simulink library "CMGlibrary"  (R2019b)
settings: Solver=VariableStepAuto  StartTime=0.0  StopTime=10.0  RelTol=1e-3
values from neighbouring files (symbols this model uses):
  angleOffset = 0 *pi/180    (= 0)    [CMGParams.m]
  CMGInertia_z = 3/4*CMGmass*(CMGr)^2    (= 0.0012)    [CMGParams.m]
  CMGmass = 1    [CMGParams.m]
  deltaLegAngleThr = 8*pi/180    (= 0.13962634016)    [CMGParams.m]
  highpassbandFreq = 10    [CMGParams.m]
  KdGammaReset = 6000    [CMGParams.m]
  KiGamma = 1    [CMGParams.m]
  KpGamma = 10    [CMGParams.m]
  KpGammaReset = 30000    [CMGParams.m]
  legAngleSpeedMax = 10    [CMGParams.m]
  lowpassbandFreq = 80    [CMGParams.m]
  maxGMangle = 60 *pi/180    (= 1.0471975512)    [CMGParams.m]
  maxGMTorque = 15    [CMGParams.m]
  maxTflywheelmotor = 1.83E-3    (= 0.00183)    [CMGParams.m]
  N = 1.5    [BodyMechParams.m]    (also in cmaes.m = size(x,1); mergeCompareEnergyCosts.m = {S.name})
  omegaRef = 2100    [CMGParams.m]
  RkneeExtendGain = 25000    [CMGParams.m]
  RkneeFlexPosGain = 6    [CMGParams.m]
  RkneeFlexSpeedGain = 6    [CMGParams.m]
  RkneeStopGain = 12000    [CMGParams.m]
  RlegAngleFilter = 100    [CMGParams.m]
  s = x(1:N-1,:).^2 + x(2:N,:).^2    [cmaes.m]
  shankLength = shankLength - ankle_height/2    (= 0.46)    [BodyMechParams.m]
  TargetLegAngleTripFlex = 2/3*pi    (= 2.09439510239)    [CMGParams.m]
  thighLength = thighLength - ankle_height/2    (= 0.46)    [BodyMechParams.m]
  tripDetectThreshold = -600    [CMGParams.m]
  X = contains(N,'compareEnergyCost') .* ~contains(N,'total') .* ~contains(N,'Total')    [mergeCompareEnergyCosts.m]
  zeroOrderHoldTs = 1/1000    (= 0.001)    [CMGParams.m]
undefined symbols (not defined in the file or in its folder): kneeExtendGain, kneeFlexPosGain, kneeFlexSpeedGain, kneeStopGain, legAngleFilter, legLengthClr, RdeltaLegAngleThr, RlegLengthClr, Y, Z
libraries: sm_lib x11, nesl_utility x11, dspfdesign x6, simulink x5, $bdroot x1, dspsigops x1
settings Model: Creator=sup-gjtimmers  LastModifiedBy=Nathan

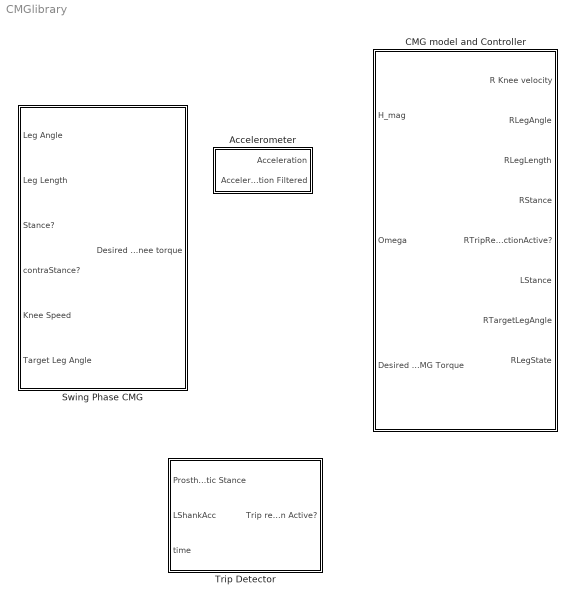
== system CMGlibrary ==
  Accelerometer : Subsystem  mask{zoh_sampletime=zeroOrderHoldTs, lowpasswp=lowpassbandFreq, highpasswp=highpassbandFreq}
      mask prompts: zoh_sampletime "Zero-order hold sample time (s)"; lowpasswp "Lowpass passband frequency (Hz)"; highpasswp "Highpass passband frequency (Hz)"
  CMG model and Controller : Subsystem  mask{KpGamma=KpGamma, KiGamma=KiGamma, legAngleFilter=RlegAngleFilter, kneeFlexSpeedGain=RkneeFlexSpeedGain, kneeFlexPosGain=RkneeFlexPosGain, kneeStopGain=RkneeStopGain, kneeExtendGain=RkneeExtendGain, legLengthClr=RlegLengthClr, TargetLegAngleTripFlex=TargetLegAngleTripFlex, deltaLegAngleThr=RdeltaLegAngleThr, legAngleSpeedMax=legAngleSpeedMax}
      mask prompts: KpGamma "Proportional Gain Gamma ( Nm/(rad/s) )"; KiGamma "Integral Gain Gamma (Nm/rad)"
  Swing Phase CMG : Subsystem  mask{legAngleFilter=legAngleFilter, kneeFlexSpeedGain=kneeFlexSpeedGain, kneeFlexPosGain=kneeFlexPosGain, kneeStopGain=kneeStopGain, kneeExtendGain=kneeExtendGain, legLengthClr=legLengthClr, TargetLegAngleTripFlex=TargetLegAngleTripFlex, deltaLegAngleThr=deltaLegAngleThr, legAngleSpeedMax=legAngleSpeedMax}
  Trip Detector : Subsystem  mask{tripThreshold=tripDetectThreshold}
      mask prompts: tripThreshold "Trip threshold (m/s^2)"

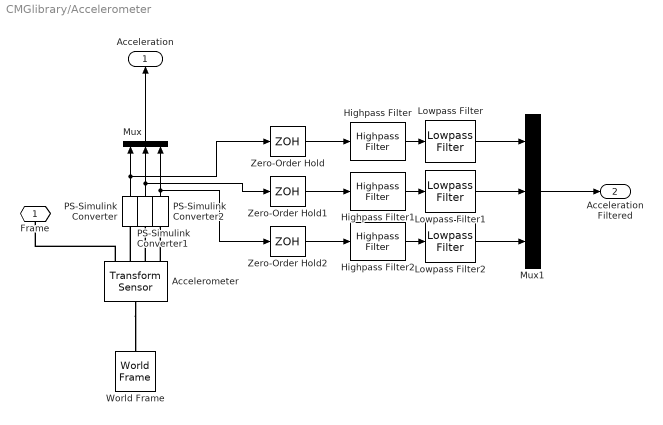
== system CMGlibrary/Accelerometer ==
  Accelerometer : sm_lib/Frames and Transforms/Transform Sensor  MeasurementFrame=World  SenseAngle=off  SenseAxis=off  SenseAngle1=off  SenseAngle2=off  SenseAngle3=off  SenseQ=off  SenseR=off  SenseOmegaX=off  SenseOmegaY=off  SenseOmegaZ=off  SenseOmega1=off  SenseOmega2=off  SenseOmega3=off  SenseQDot=off  SenseRDot=off  SenseAlphaX=off  SenseAlphaY=off  SenseAlphaZ=off  SenseAlpha1=off  SenseAlpha2=off  SenseAlpha3=off  SenseQDDot=off  SenseRDDot=off  SenseX=off  SenseY=off  SenseZ=off  SenseRad=off  SenseAzim=off  SenseDist=off  SenseInc=off  SenseXDot=off  SenseYDot=off  SenseZDot=off  SenseRadDot=off  SenseAzimDot=off  SenseDistDot=off  SenseIncDot=off  SenseXDDot=on  SenseYDDot=on  SenseZDDot=on  SenseRadDDot=off  SenseAzimDDot=off  SenseDistDDot=off  SenseIncDDot=off
  Highpass Filter : dspfdesign/Highpass Filter  FilterType=IIR  DesignForMinimumOrder=off  FilterOrder=2  StopbandFrequency=2.5  PassbandFrequency=highpasswp  StopbandAttenuation=60  PassbandRipple=0.1  InheritSampleRate=on  SampleRate=1000  SimulateUsing=Interpreted execution  roundingMode=Floor  coeffsDataTypeStr=fixdt(1,16)
      settings: SourceProductName=DSP System Toolbox
  Highpass Filter1 : dspfdesign/Highpass Filter  FilterType=IIR  DesignForMinimumOrder=off  FilterOrder=2  StopbandFrequency=2.5  PassbandFrequency=highpasswp  StopbandAttenuation=60  PassbandRipple=0.1  InheritSampleRate=on  SampleRate=1000  SimulateUsing=Interpreted execution  roundingMode=Floor  coeffsDataTypeStr=fixdt(1,16)
      settings: SourceProductName=DSP System Toolbox
  Highpass Filter2 : dspfdesign/Highpass Filter  FilterType=IIR  DesignForMinimumOrder=off  FilterOrder=2  StopbandFrequency=2.5  PassbandFrequency=highpasswp  StopbandAttenuation=60  PassbandRipple=0.1  InheritSampleRate=on  SampleRate=1000  SimulateUsing=Interpreted execution  roundingMode=Floor  coeffsDataTypeStr=fixdt(1,16)
      settings: SourceProductName=DSP System Toolbox
  Lowpass Filter : dspfdesign/Lowpass Filter  FilterType=IIR  DesignForMinimumOrder=off  FilterOrder=2  PassbandFrequency=lowpasswp  StopbandFrequency=41  PassbandRipple=0.2  StopbandAttenuation=80  InheritSampleRate=on  SampleRate=1000  SimulateUsing=Interpreted execution  roundingMode=Floor  coeffsDataTypeStr=fixdt(1,16)
  Lowpass Filter1 : dspfdesign/Lowpass Filter  FilterType=IIR  DesignForMinimumOrder=off  FilterOrder=2  PassbandFrequency=lowpasswp  StopbandFrequency=41  PassbandRipple=0.2  StopbandAttenuation=80  InheritSampleRate=on  SampleRate=1000  SimulateUsing=Interpreted execution  roundingMode=Floor  coeffsDataTypeStr=fixdt(1,16)
  Lowpass Filter2 : dspfdesign/Lowpass Filter  FilterType=IIR  DesignForMinimumOrder=off  FilterOrder=2  PassbandFrequency=lowpasswp  StopbandFrequency=41  PassbandRipple=0.2  StopbandAttenuation=80  InheritSampleRate=on  SampleRate=1000  SimulateUsing=Interpreted execution  roundingMode=Floor  coeffsDataTypeStr=fixdt(1,16)
  Mux : Mux  Inputs=3
  Mux1 : Mux  Inputs=3
  PS-Simulink Converter : nesl_utility/PS-Simulink Converter  PhysicalDomain=network_engine_domain  SubClassName=ps_output  LeftPortType=input  RightPortType=output  PseudoPeriodic=off  Frequencies=[]  Unit=m/s^ 2  AffineConversion=off
  PS-Simulink Converter1 : nesl_utility/PS-Simulink Converter  PhysicalDomain=network_engine_domain  SubClassName=ps_output  LeftPortType=input  RightPortType=output  PseudoPeriodic=off  Frequencies=[]  Unit=m/s^ 2  AffineConversion=off
  PS-Simulink Converter2 : nesl_utility/PS-Simulink Converter  PhysicalDomain=network_engine_domain  SubClassName=ps_output  LeftPortType=input  RightPortType=output  PseudoPeriodic=off  Frequencies=[]  Unit=m/s^ 2  AffineConversion=off
  World Frame : sm_lib/Frames and Transforms/World Frame
  Zero-Order Hold : ZeroOrderHold  SampleTime=zoh_sampletime
  Zero-Order Hold1 : ZeroOrderHold  SampleTime=zoh_sampletime
  Zero-Order Hold2 : ZeroOrderHold  SampleTime=zoh_sampletime
  Frame : PMIOPort  Side=Left
  Acceleration : Outport
  Acceleration Filtered : Outport  Port=2
  wires:
  PS-Simulink Converter1/1 -> Zero-Order Hold1/1, Mux/2
  PS-Simulink Converter/1 -> Mux/1, Zero-Order Hold/1
  Mux/1 -> Acceleration/1
  PS-Simulink Converter2/1 -> Zero-Order Hold2/1, Mux/3
  Zero-Order Hold/1 -> Highpass Filter/1
  Highpass Filter/1 -> Lowpass Filter/1
  Highpass Filter1/1 -> Lowpass Filter1/1
  Zero-Order Hold1/1 -> Highpass Filter1/1
  Zero-Order Hold2/1 -> Highpass Filter2/1
  Highpass Filter2/1 -> Lowpass Filter2/1
  Lowpass Filter2/1 -> Mux1/3
  Lowpass Filter1/1 -> Mux1/2
  Lowpass Filter/1 -> Mux1/1
  Mux1/1 -> Acceleration Filtered/1
  connections:
  Accelerometer/LConn1 -- World Frame/RConn1
  Accelerometer/RConn3 -- PS-Simulink Converter1/LConn1
  Accelerometer/RConn1 -- Frame/RConn1
  Accelerometer/RConn2 -- PS-Simulink Converter/LConn1
  Accelerometer/RConn4 -- PS-Simulink Converter2/LConn1

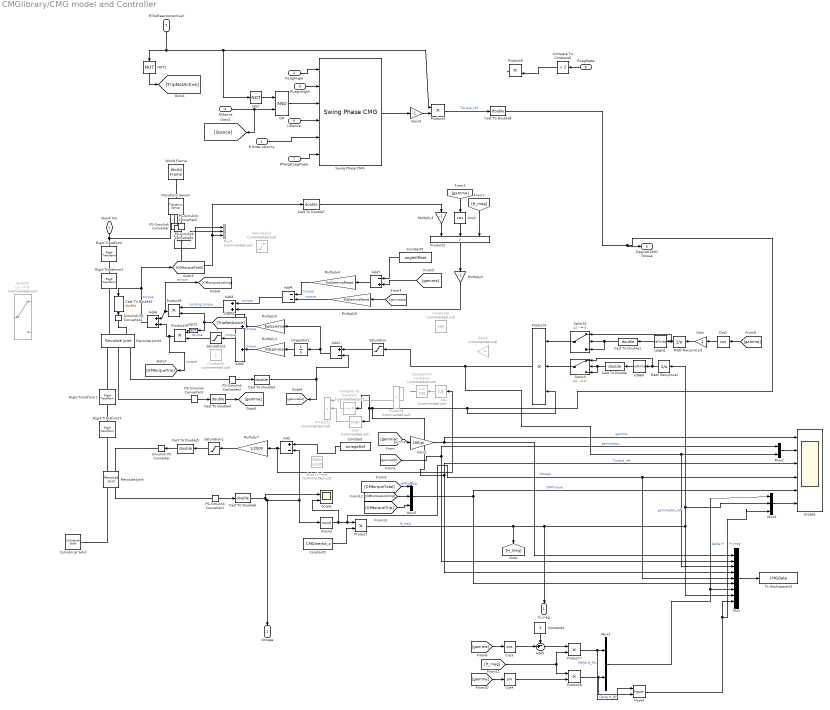
== system CMGlibrary/CMG model and Controller ==
  R Knee velocity : Inport
  RLegAngle : Inport  Port=2
  RLegLength : Inport  Port=3
  RStance : Inport  Port=4
  RTripReactionActive? : Inport  Port=5
  LStance : Inport  Port=6
  RTargetLegAngle : Inport  Port=7
  RLegState : Inport  Port=8
  Abs : Abs  Commented=on  ZeroCross=off
  Add : Sum  Inputs=+-
  Add1 : Sum  Inputs=+-
  Add2 : Sum
  Add3 : Sum
  Add4 : Sum  Inputs=--
  Add5 : Sum  Inputs=-+|
  Add6 : Sum
  Add7 : Sum  Inputs=-+
  Cast To Double{,1..8} (9 alike) : DataTypeConversion  OutDataTypeStr=double  LockScale=on
  Compare To Constant : simulink/Logic and Bit Operations/Compare To Constant  Commented=on  relop=~=  const=0  OutDataTypeStr=boolean  ZeroCross=off
  Compare To Constant1 : simulink/Logic and Bit Operations/Compare To Constant  Commented=on  relop=<=  const=100  OutDataTypeStr=boolean  ZeroCross=off
  Compare To Constant2 : simulink/Logic and Bit Operations/Compare To Constant  relop=<  const=2  OutDataTypeStr=boolean
  Constant : Constant  Value=omegaRef
  Constant1 : Constant  Value=CMGInertia_z
  Constant2 : Constant  Commented=on  Value=150
  Constant3 : Constant  Commented=on
  Constant4 : Constant
  Constant5 : Constant  Value=angleOffset
  Cos1 : Trigonometry  Operator=cos  OutputSignalType=real
  Cos2 : Trigonometry  Operator=cos  OutputSignalType=real
  Cos3 : Trigonometry  Operator=cos  OutputSignalType=real
  Cos4 : Trigonometry  OutputSignalType=real
  Cylindrical Solid : sm_lib/Body Elements/Cylindrical Solid  GraphicAmbientColor=[0.15 0.15 0.15 1.0]  BasedOnType=Mass  CenterOfMass=[0 0 0]  CenterOfMassUnits=m  GraphicDiffuseColor=[0.5 0.5 0.5]  CylinderLength=CMGt  CylinderLengthUnits=m  CylinderRadius=CMGr  CylinderRadiusUnits=m  Density=1000000  DensityUnits=kg/m^3  DoExposeReferenceFrame=on  GraphicEmissiveColor=[0.0 0.0 0.0 1.0]  ExportEntireGeometry=off  SerializedFrames=<Frames/>  MarkerShape=Sphere  MarkerSize=10  GraphicType=FromGeometry  InertiaType=Custom  Mass=CMGmass  MassUnits=kg  MomentsOfInertia=CMGInertia  MomentsOfInertiaUnits=kg*m^2  GraphicOpacity=1.0  ProductsOfInertia=[0 0 0]  ProductsOfInertiaUnits=kg*m^2  GraphicShininess=75  GraphicSpecularColor=[0.5 0.5 0.5 1.0]  GraphicVisPropType=SimpleVisualProperties
  Gain : Gain
  Gain1 : Gain  Commented=on  Gain=4
  Gain2 : Gain  Gain=180/pi
  Gain3 : Gain  Gain=-1
  Hypot : Math  Operator=hypot  SignedPower=off  SaturateOnIntegerOverflow=on
  Integrator1 : Integrator
  IsNaN : RelationalOperator  Operator=isFinite  OutDataTypeStr=boolean  RndMeth=Simplest
  IsNaN1 : RelationalOperator  Operator=isFinite  OutDataTypeStr=boolean  RndMeth=Simplest
  Math Reciprocal : Math  Operator=reciprocal  SaturateOnIntegerOverflow=on
  Math Reciprocal1 : Math  Operator=reciprocal  SaturateOnIntegerOverflow=on
  Multiply1 : Gain  Gain=KiGamma
  Multiply2 : Gain  Gain=-1
  Multiply3 : Gain  Gain=-1
  Multiply4 : Gain  Gain=KpGammaReset
  Multiply5 : Gain  Gain=KpGamma
  Multiply6 : Gain  Gain=KdGammaReset
  Multiply7 : Gain  Gain=1/2000
  Mux : Mux  Inputs=9
  Mux1 : Mux  Commented=on  Inputs=3
  Mux2 : Mux  Inputs=2
  Mux3 : Mux  Inputs=2
  Mux4 : Mux  Inputs=3
  Mux5 : Mux  Inputs=3
  NOT : Logic  Operator=NOT  IconShape=distinctive  AllPortsSameDT=off  OutDataTypeStr=boolean
  NOT1 : Logic  Operator=NOT  IconShape=distinctive  AllPortsSameDT=off  OutDataTypeStr=boolean
  NOT2 : Logic  Operator=NOT  IconShape=distinctive  AllPortsSameDT=off  OutDataTypeStr=boolean
  OR : Logic  AllPortsSameDT=off  OutDataTypeStr=boolean
  PS-Simulink Converter{,1,4..5} (4 alike) : nesl_utility/PS-Simulink Converter  PhysicalDomain=network_engine_domain  SubClassName=ps_output  LeftPortType=input  RightPortType=output  PseudoPeriodic=off  Frequencies=[]  Unit=inherit  AffineConversion=off
  PS-Simulink Converter2 : nesl_utility/PS-Simulink Converter  PhysicalDomain=network_engine_domain  SubClassName=ps_output  LeftPortType=input  RightPortType=output  PseudoPeriodic=off  Frequencies=[]  Unit=rad/s  AffineConversion=off
  PS-Simulink Converter3 : nesl_utility/PS-Simulink Converter  PhysicalDomain=network_engine_domain  SubClassName=ps_output  LeftPortType=input  RightPortType=output  PseudoPeriodic=off  Frequencies=[]  Unit=rad  AffineConversion=off
  Product{,5..10} (7 alike) : Product
  Product1 : Product  Commented=on  Inputs=3
  Product2 : Product  Inputs=3
  Product3 : Product  Commented=on
  Product4 : Product  Inputs=***
  Rate Limiter : RateLimiter  Commented=on  RisingSlewLimit=100000  FallingSlewLimit=-100000  SampleTimeMode=inherited
  Revolute Joint : sm_lib/Joints/Revolute Joint  JointMode=Normal  SenseConstraintForce=off  SenseConstraintForceX=off  SenseConstraintForceY=off  SenseConstraintForceZ=off  SenseConstraintTorque=off  SenseConstraintTorqueX=off  SenseConstraintTorqueY=off  SenseConstraintTorqueZ=off  SenseTotalForce=off  SenseTotalForceX=off  SenseTotalForceY=off  SenseTotalForceZ=off  SenseTotalTorque=off  SenseTotalTorqueX=off  SenseTotalTorqueY=off  SenseTotalTorqueZ=off  CompositeWrenchDir=FollowerOnBase  CompositeWrenchFrame=BaseFrame  EquilibriumPosition=0  EquilibriumPositionUnits=deg  SpringStiffness=0  SpringStiffnessUnits=N*m/deg  DampingCoefficient=0  DampingCoefficientUnits=N*m/(deg/s)  TorqueActuationMode=InputTorque  MotionActuationMode=ComputedMotion  SensePosition=off  SenseVelocity=on  SenseAcceleration=off  SenseTorqueForce=off  SenseLowerLimitTorqueForce=off  SenseUpperLimitTorqueForce=off  LowerLimitSpecify=off  LowerLimitBound=-90  LowerLimitBoundUnits=deg  LowerLimitStiffness=1e4  LowerLimitStiffnessUnits=N*m/deg  LowerLimitDamping=10  LowerLimitDampingUnits=N*m/(deg/s)  LowerLimitTransitionRegionWidth=0.1  LowerLimitTransitionRegionWidthUnits=deg  UpperLimitSpecify=off  UpperLimitBound=90  UpperLimitBoundUnits=deg  UpperLimitStiffness=1e4  UpperLimitStiffnessUnits=N*m/deg  UpperLimitDamping=10  UpperLimitDampingUnits=N*m/(deg/s)  UpperLimitTransitionRegionWidth=0.1  UpperLimitTransitionRegionWidthUnits=deg  PositionTargetSpecify=off  PositionTargetPriority=High  PositionTargetValue=0  PositionTargetValueUnits=deg  VelocityTargetSpecify=on  VelocityTargetPriority=High  VelocityTargetValue=omegaRef  VelocityTargetValueUnits=rad/s
  Revolute Joint2 : sm_lib/Joints/Revolute Joint  JointMode=Normal  SenseConstraintForce=off  SenseConstraintForceX=off  SenseConstraintForceY=off  SenseConstraintForceZ=off  SenseConstraintTorque=off  SenseConstraintTorqueX=off  SenseConstraintTorqueY=off  SenseConstraintTorqueZ=off  SenseTotalForce=off  SenseTotalForceX=off  SenseTotalForceY=off  SenseTotalForceZ=off  SenseTotalTorque=off  SenseTotalTorqueX=off  SenseTotalTorqueY=off  SenseTotalTorqueZ=off  CompositeWrenchDir=FollowerOnBase  CompositeWrenchFrame=BaseFrame  EquilibriumPosition=0  EquilibriumPositionUnits=deg  SpringStiffness=0  SpringStiffnessUnits=N*m/deg  DampingCoefficient=0  DampingCoefficientUnits=N*m/(deg/s)  TorqueActuationMode=InputTorque  MotionActuationMode=ComputedMotion  SensePosition=on  SenseVelocity=on  SenseAcceleration=off  SenseTorqueForce=off  SenseLowerLimitTorqueForce=off  SenseUpperLimitTorqueForce=off  LowerLimitSpecify=on  LowerLimitBound=-maxGMangle  LowerLimitBoundUnits=rad  LowerLimitStiffness=1e4  LowerLimitStiffnessUnits=N*m/deg  LowerLimitDamping=10  LowerLimitDampingUnits=N*m/(deg/s)  LowerLimitTransitionRegionWidth=0.1  LowerLimitTransitionRegionWidthUnits=deg  UpperLimitSpecify=on  UpperLimitBound=maxGMangle  UpperLimitBoundUnits=rad  UpperLimitStiffness=1e4  UpperLimitStiffnessUnits=N*m/deg  UpperLimitDamping=10  UpperLimitDampingUnits=N*m/(deg/s)  UpperLimitTransitionRegionWidth=0.1  UpperLimitTransitionRegionWidthUnits=deg  PositionTargetSpecify=on  PositionTargetPriority=High  PositionTargetValue=angleOffset  PositionTargetValueUnits=rad  VelocityTargetSpecify=on  VelocityTargetPriority=High  VelocityTargetValue=0  VelocityTargetValueUnits=rad/s
  Rigid Transform : sm_lib/Frames and Transforms/Rigid Transform  TranslationMethod=Cartesian  TranslationStandardOffset=0  TranslationLengthUnit=m  TranslationStandardAxis=+Z  TranslationCartesianOffset=[0 -0.015 0]  TranslationROffset=0  TranslationROffsetUnits=m  TranslationZOffset=0  TranslationZOffsetUnits=m  TranslationThetaOffset=0  TranslationThetaOffsetUnits=deg  RotationMethod=None  RotationAngleUnits=deg  RotationStandardAxis=+Z  RotationAngle=0.0  RotationArbitraryAxis=[0 0 1]  FollAlignAxisA=+X  BaseAlignAxisA=+Y  FollAlignAxisB=+Y  BaseAlignAxisB=+Z  RotationSequenceAxes=FollowerAxes  RotationSequence=XYX  RotationSequenceAngles=[0 0 0]  RotationSequenceAnglesUnits=deg  RotationMatrix=[1 0 0; 0 1 0; 0 0 1]
  Rigid Transform1 : sm_lib/Frames and Transforms/Rigid Transform  TranslationMethod=Cartesian  TranslationStandardOffset=0  TranslationLengthUnit=m  TranslationStandardAxis=+Z  TranslationCartesianOffset=[0 0 0.04]  TranslationROffset=0  TranslationROffsetUnits=m  TranslationZOffset=0  TranslationZOffsetUnits=m  TranslationThetaOffset=0  TranslationThetaOffsetUnits=deg  RotationMethod=None  RotationAngleUnits=deg  RotationStandardAxis=+Z  RotationAngle=0.0  RotationArbitraryAxis=[0 0 1]  FollAlignAxisA=+X  BaseAlignAxisA=+Y  FollAlignAxisB=+Y  BaseAlignAxisB=+Z  RotationSequenceAxes=FollowerAxes  RotationSequence=XYX  RotationSequenceAngles=[0 0 0]  RotationSequenceAnglesUnits=deg  RotationMatrix=[1 0 0; 0 1 0; 0 0 1]
  Rigid Transform2 : sm_lib/Frames and Transforms/Rigid Transform  TranslationMethod=None  TranslationStandardOffset=0  TranslationLengthUnit=m  TranslationStandardAxis=+Z  TranslationCartesianOffset=[0 0 0]  TranslationROffset=0  TranslationROffsetUnits=m  TranslationZOffset=0  TranslationZOffsetUnits=m  TranslationThetaOffset=0  TranslationThetaOffsetUnits=deg  RotationMethod=AlignedAxes  RotationAngleUnits=deg  RotationStandardAxis=+Z  RotationAngle=0.0  RotationArbitraryAxis=[0 0 1]  FollAlignAxisA=+Z  BaseAlignAxisA=+X  FollAlignAxisB=+Y  BaseAlignAxisB=+Y  RotationSequenceAxes=FollowerAxes  RotationSequence=XYX  RotationSequenceAngles=[0 0 0]  RotationSequenceAnglesUnits=deg  RotationMatrix=[1 0 0; 0 1 0; 0 0 1]
  Rigid Transform5 : sm_lib/Frames and Transforms/Rigid Transform  TranslationMethod=None  TranslationStandardOffset=0  TranslationLengthUnit=m  TranslationStandardAxis=+Z  TranslationCartesianOffset=[0 0 0.02]  TranslationROffset=0  TranslationROffsetUnits=m  TranslationZOffset=0  TranslationZOffsetUnits=m  TranslationThetaOffset=0  TranslationThetaOffsetUnits=deg  RotationMethod=AlignedAxes  RotationAngleUnits=deg  RotationStandardAxis=+Z  RotationAngle=0.0  RotationArbitraryAxis=[0 0 1]  FollAlignAxisA=+Z  BaseAlignAxisA=-Y  FollAlignAxisB=+X  BaseAlignAxisB=+Z  RotationSequenceAxes=FollowerAxes  RotationSequence=XYX  RotationSequenceAngles=[0 0 0]  RotationSequenceAnglesUnits=deg  RotationMatrix=[1 0 0; 0 1 0; 0 0 1]
  Round : Rounding  Operator=round
  Saturation : Saturate  UpperLimit=500  LowerLimit=-500
  Saturation1 : Saturate  UpperLimit=maxTflywheelmotor  LowerLimit=-maxTflywheelmotor
  Saturation2 : Saturate  UpperLimit=maxGMTorque  LowerLimit=-maxGMTorque
  Saturation3 : Saturate  Commented=on  UpperLimit=2  LowerLimit=-2  ZeroCross=off
  Scope : Scope  NumInputPorts=2
  Scope1 : Scope  NumInputPorts=6
  Sign : Signum  Commented=on  ZeroCross=off
  Simulink-PS Converter : nesl_utility/Simulink-PS Converter  PhysicalDomain=network_engine_domain  SubClassName=ps_input  LeftPortType=input  RightPortType=output  PseudoPeriodic=off  Frequencies=[]  NoiseDistribution=none  NoiseParameters=[]  Unit=1  AffineConversion=off  FilteringAndDerivatives=provide  SimscapeFilterOrder=1  InputFilterTimeConstant=0.001  UdotUserProvided=0
  Simulink-PS Converter1 : nesl_utility/Simulink-PS Converter  PhysicalDomain=network_engine_domain  SubClassName=ps_input  LeftPortType=input  RightPortType=output  PseudoPeriodic=off  Frequencies=[]  NoiseDistribution=none  NoiseParameters=[]  Unit=1  AffineConversion=off  FilteringAndDerivatives=provide  SimscapeFilterOrder=1  InputFilterTimeConstant=0.001  UdotUserProvided=0
  Swing Phase CMG : $bdroot/Swing Phase CMG  legAngleFilter=RlegAngleFilter  kneeFlexSpeedGain=kneeFlexSpeedGain  kneeFlexPosGain=kneeFlexPosGain  kneeStopGain=RkneeStopGain  kneeExtendGain=RkneeExtendGain  legLengthClr=RlegLengthClr  TargetLegAngleTripFlex=TargetLegAngleTripFlex  deltaLegAngleThr=deltaLegAngleThr  legAngleSpeedMax=legAngleSpeedMax
  Switch : Switch  Criteria=u2 ~= 0
  Switch1 : Switch  Criteria=u2 ~= 0
  Switch2 : Switch  Commented=on  Criteria=u2 ~= 0
  To Workspace13 : ToWorkspace  VariableName=CMGData  SaveFormat=Structure With Time  SampleTime=-1
  Transform Sensor : sm_lib/Frames and Transforms/Transform Sensor  MeasurementFrame=Follower  SenseAngle=off  SenseAxis=off  SenseAngle1=off  SenseAngle2=off  SenseAngle3=off  SenseQ=off  SenseR=off  SenseOmegaX=on  SenseOmegaY=on  SenseOmegaZ=on  SenseOmega1=off  SenseOmega2=off  SenseOmega3=off  SenseQDot=off  SenseRDot=off  SenseAlphaX=off  SenseAlphaY=off  SenseAlphaZ=off  SenseAlpha1=off  SenseAlpha2=off  SenseAlpha3=off  SenseQDDot=off  SenseRDDot=off  SenseX=off  SenseY=off  SenseZ=off  SenseRad=off  SenseAzim=off  SenseDist=off  SenseInc=off  SenseXDot=off  SenseYDot=off  SenseZDot=off  SenseRadDot=off  SenseAzimDot=off  SenseDistDot=off  SenseIncDot=off  SenseXDDot=off  SenseYDDot=off  SenseZDDot=off  SenseRadDDot=off  SenseAzimDDot=off  SenseDistDDot=off  SenseIncDDot=off
  World Frame : sm_lib/Frames and Transforms/World Frame
  Shank CG : PMIOPort  Side=Left
  H_mag : Outport
  Omega : Outport  Port=2
  Desired CMG Torque : Outport  Port=3
  wires:
  RTargetLegAngle/1 -> Swing Phase CMG/6
  IsNaN1/1 -> Cast To Double1/1
  Gain3/1 -> Product5/2
  LStance/1 -> Swing Phase CMG/4
  RStance/1 -> [Stance], OR/2
  R Knee velocity/1 -> Swing Phase CMG/5
  IsNaN/1 -> Cast To Double/1
  Switch1/1 -> Product4/1
  Mux/1 -> To Workspace13/1
  Gain/1 -> Math Reciprocal1/1
  [gamma] -> Cos1/1
  Math Reciprocal1/1 -> Switch1/1, IsNaN1/1
  Cast To Double/1 -> Switch/2, Switch/3
  Product5/1 -> Cast To Double8/1  "Torque_ref"
  [gammadot] -> Mux2/1, Mux/2  "gammadot"
  PS-Simulink Converter1/1 -> Cast To Double6/1
  Product4/1 -> Mux/3, Mux2/2, Saturation/1  "gammadot_ref"
  [gamma] -> Cos3/1
  Multiply6/1 -> Add4/2  "torque"
  Abs/1 -> Compare To Constant1/1
  Product8/1 -> Hypot/2, Mux3/2  "Delta H_AP"
  Constant4/1 -> Add5/1
  Mux2/1 -> Scope1/2
  Cos4/1 -> Product8/2
  Mux4/1 -> Scope1/6
  RLegState/1 -> Compare To Constant2/1
  Saturation/1 -> Add1/1
  Round/1 -> Scope/2, Mux/5, Scope1/4, Product/1  "Omega"
  Cast To Double1/1 -> Switch1/3, Switch1/2
  Product/1 -> [H_mag], Mux/8, Mux4/2, Math Reciprocal/1, H_mag/1  "H_mag"
  Swing Phase CMG/1 -> Gain3/1
  Mux5/1 -> Mux/6, Scope1/5  "GMTorque"
  [TripNotActive] -> Product9/2, NOT2/1
  Compare To Constant2/1 -> Product6/2
  Multiply2/1 -> Add3/2
  PS-Simulink Converter/1 -> Mux1/1
  Multiply3/1 -> Product2/1
  Constant1/1 -> Product/2
  Cos2/1 -> Product2/2
  NOT1/1 -> [TripNotActive]
  Add2/1 -> Saturation2/1  "torque"
  Math Reciprocal/1 -> IsNaN/1, Switch/1
  RLegAngle/1 -> Swing Phase CMG/1
  OR/1 -> Swing Phase CMG/3
  [H_mag] -> Product2/3
  Integrator1/1 -> Multiply1/1
  [gamma] -> Cos2/1
  Saturation1/1 -> Cast To Double5/1
  Multiply5/1 -> Add2/1  "torque"
  Product6/1 -> ?
  Compare To Constant1/1 -> ?
  Hypot/1 -> Mux4/3, Mux/9  "H_mag-"
  [GMtorqueLocking] -> Mux5/2
  Add3/1 -> Product9/1  "Locking torque"
  PS-Simulink Converter3/1 -> Cast To Double4/1
  PS-Simulink Converter5/1 -> Mux1/3, Cast To Double7/1
  Saturation2/1 -> Product10/2  "torque"
  [gamma] -> Cos4/1
  Multiply4/1 -> Add4/1  "torque"
  Cast To Double8/1 -> Desired CMG Torque/1, Mux/4, Scope1/3, Compare To Constant/1, Sign/1, Product4/3  "Torque_ref"
  Add1/1 -> Multiply5/1, Integrator1/1
  PS-Simulink Converter4/1 -> Mux1/2
  Multiply7/1 -> Saturation1/1
  Sign/1 -> Product1/2
  Product7/1 -> Hypot/1, Mux3/1  "Delta H_ML"
  RTripReactionActive?/1 -> Product5/1, NOT/1, NOT1/1
  Add5/1 -> Product7/1
  Cos1/1 -> Gain/1
  [gamma] -> Add7/2
  Gain2/1 -> Scope1/1, Mux/1  "gamma"
  Cast To Double6/1 -> Omega/1, Add/2, Round/1, Scope/1
  Cast To Double5/1 -> Simulink-PS Converter/1
  [gammadot] -> Multiply6/1
  [GMtorqueTotal] -> Mux5/1  "GMTorque"
  Cast To Double4/1 -> [gamma]
  RLegLength/1 -> Swing Phase CMG/2
  Product9/1 -> [GMtorqueLocking], Add6/1  "torque"
  Product2/1 -> Multiply2/1
  NOT2/1 -> Product10/1
  NOT/1 -> OR/1
  Multiply1/1 -> Add2/2  "torque"
  Switch/1 -> Product4/2
  [H_mag] -> Product7/2, Product8/1
  Cast To Double2/1 -> Simulink-PS Converter1/1
  PS-Simulink Converter2/1 -> Cast To Double3/1
  Compare To Constant/1 -> Product1/1
  Cos3/1 -> Add5/2
  Product10/1 -> [GMtorqueTrip], Add6/2  "torque"
  Add6/1 -> Cast To Double2/1, [GMtorqueTotal]  "torque"
  [gamma] -> Gain2/1  "gamma"
  Cast To Double3/1 -> Add1/2, [gammadot]
  Cast To Double7/1 -> Multiply3/1
  [GMtorqueTrip] -> Mux5/3
  Add4/1 -> Add3/1  "torque"
  Constant/1 -> Add/1
  Add/1 -> Multiply7/1, Abs/1
  Mux3/1 -> Mux4/1, Mux/7  "Delta H"
  Add7/1 -> Multiply4/1
  Constant5/1 -> Add7/1
  connections:
  Shank CG/RConn1 -- Rigid Transform/LConn1 -- Transform Sensor/RConn1
  Rigid Transform1/RConn1 -- Rigid Transform5/LConn1
  Revolute Joint2/LConn1 -- Rigid Transform2/RConn1
  PS-Simulink Converter/LConn1 -- Transform Sensor/RConn2
  Revolute Joint2/RConn3 -- PS-Simulink Converter2/LConn1
  Simulink-PS Converter1/RConn1 -- Revolute Joint2/LConn2
  Revolute Joint/RConn2 -- PS-Simulink Converter1/LConn1
  Rigid Transform2/LConn1 -- Rigid Transform/RConn1
  World Frame/RConn1 -- Transform Sensor/LConn1
  PS-Simulink Converter5/LConn1 -- Transform Sensor/RConn4
  Revolute Joint2/RConn1 -- Rigid Transform1/LConn1
  Revolute Joint/LConn2 -- Simulink-PS Converter/RConn1
  Revolute Joint/LConn1 -- Rigid Transform5/RConn1
  PS-Simulink Converter4/LConn1 -- Transform Sensor/RConn3
  Cylindrical Solid/RConn1 -- Revolute Joint/RConn1
  PS-Simulink Converter3/LConn1 -- Revolute Joint2/RConn2

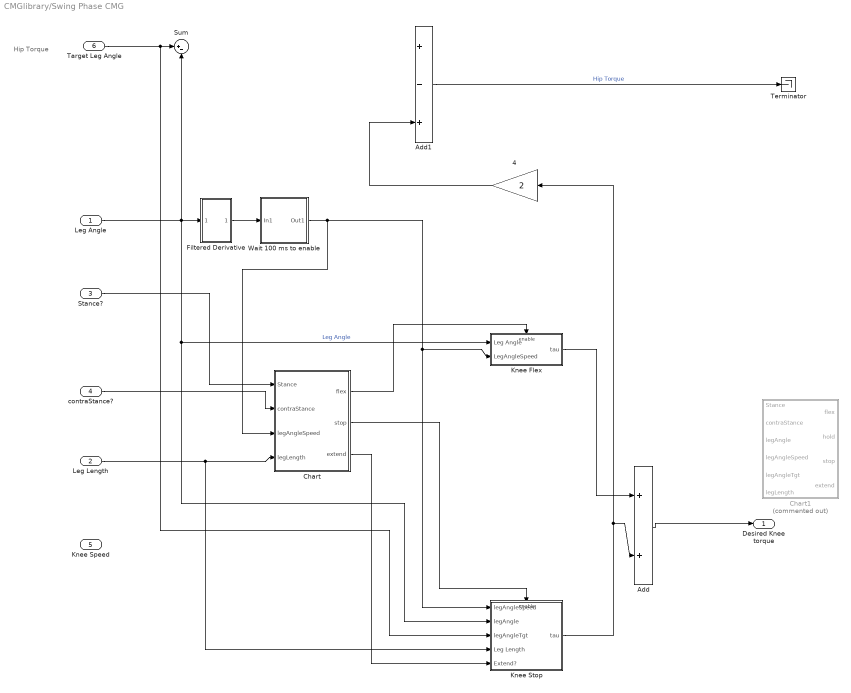
== system CMGlibrary/Swing Phase CMG ==
  note: Hip Torque
  Leg Angle : Inport
  Leg Length : Inport  Port=2
  Stance? : Inport  Port=3
  contraStance? : Inport  Port=4
  Knee Speed : Inport  Port=5
  Target Leg Angle : Inport  Port=6
  " 4" : Gain  Gain=2
  Add : Sum
  Add1 : Sum  Inputs=+-+
  Chart : Stateflow chart  TreatAsAtomicUnit=on
  Chart1 : Stateflow chart  Commented=on  TreatAsAtomicUnit=on
  Filtered Derivative : Subsystem
  Knee Flex : Subsystem  TreatAsAtomicUnit=on
  Knee Stop : Subsystem  TreatAsAtomicUnit=on
  Sum : Sum  Inputs=|+-
  Terminator : Terminator
  Wait 100 ms to enable : Subsystem
  Desired Knee torque : Outport
  wires:
  Wait 100 ms to enable/1(Out1) -> Chart/3(legAngleSpeed), Knee Stop/1(legAngleSpeed), Knee Flex/2(LegAngleSpeed)
  Filtered Derivative/1(Out1) -> Wait 100 ms to enable/1(In1)
  Target Leg Angle/1 -> Sum/1, Knee Stop/3(legAngleTgt)
  ? -> Add1/2
  ? -> Add1/1
  Leg Angle/1 -> Filtered Derivative/1(In1), Knee Flex/1(Leg Angle), Knee Stop/2(legAngle), Sum/2  "Leg Angle"
  Knee Flex/1(tau) -> Add/1
  " 4"/1 -> Add1/3
  Chart/1(flex) -> Knee Flex/Enable
  Chart/2(stop) -> Knee Stop/Enable
  Chart/3(extend) -> Knee Stop/5(Extend?)
  Stance?/1 -> Chart/1(Stance)
  contraStance?/1 -> Chart/2(contraStance)
  Leg Length/1 -> Chart/4(legLength), Knee Stop/4(Leg Length)
  Add1/1 -> Terminator/1  "Hip Torque"
  Add/1 -> Desired Knee torque/1
  Knee Stop/1(tau) -> Add/2, " 4"/1

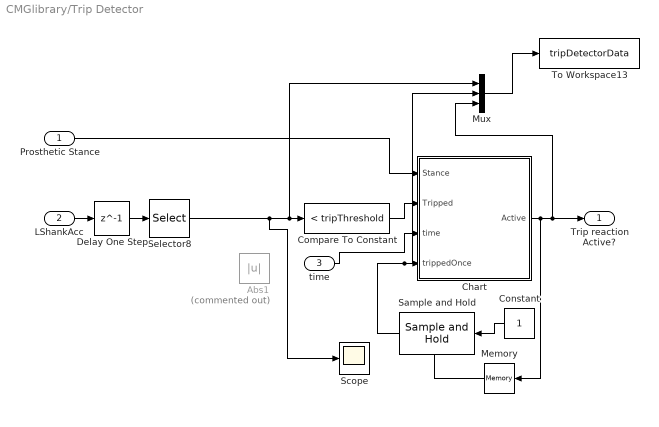
== system CMGlibrary/Trip Detector ==
  Prosthetic Stance : Inport
  LShankAcc : Inport  Port=2
  time : Inport  Port=3
  Abs1 : Abs  Commented=on
  Chart : Stateflow chart  TreatAsAtomicUnit=on
  Compare To Constant : simulink/Logic and Bit Operations/Compare To Constant  relop=<  const=tripThreshold  OutDataTypeStr=boolean
  Constant : Constant
  Delay One Step : Delay  DelayLength=1
  Memory : Memory  InheritSampleTime=on  LinearizeMemory=on  LinearizeAsDelay=on
  Mux : Mux  Inputs=3
  Sample and Hold : dspsigops/Sample and Hold  trig=Rising edge  initCond=0  latchinput=off
  Scope : Scope
  Selector8 : Selector  InputPortWidth=3  IndexOptions=Index vector (dialog)  Indices=[1]  OutputSizes=1
  To Workspace13 : ToWorkspace  VariableName=tripDetectorData  SaveFormat=Structure With Time  SampleTime=-1
  Trip reaction Active? : Outport
  wires:
  Constant/1 -> Sample and Hold/1
  Delay One Step/1 -> Selector8/1
  Sample and Hold/1 -> Mux/2, Chart/4(trippedOnce)
  Memory/1 -> Sample and Hold/Trigger
  time/1 -> Chart/3(time)
  Compare To Constant/1 -> Chart/2(Tripped)
  Selector8/1 -> Scope/1, Mux/1, Compare To Constant/1
  LShankAcc/1 -> Delay One Step/1
  Prosthetic Stance/1 -> Chart/1(Stance)
  Chart/1(Active) -> Mux/3, Trip reaction Active?/1, Memory/1
  Mux/1 -> To Workspace13/1

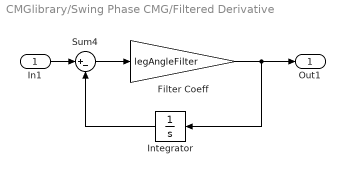
== system CMGlibrary/Swing Phase CMG/Filtered Derivative ==
  In1 : Inport
  Filter Coeff : Gain  Gain=legAngleFilter
  Integrator : Integrator
  Sum4 : Sum  Inputs=|+-
  Out1 : Outport
  wires:
  In1/1 -> Sum4/1
  Filter Coeff/1 -> Out1/1, Integrator/1
  Sum4/1 -> Filter Coeff/1
  Integrator/1 -> Sum4/2

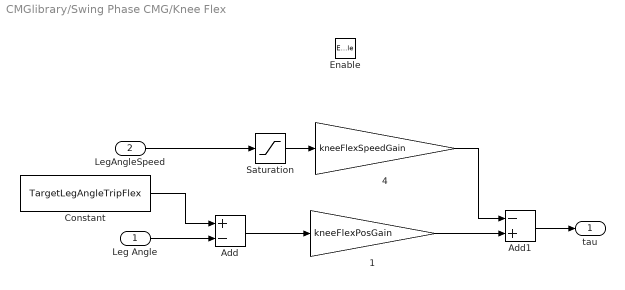
== system CMGlibrary/Swing Phase CMG/Knee Flex ==
  Leg Angle : Inport
  LegAngleSpeed : Inport  Port=2
  Enable : EnablePort  StatesWhenEnabling=reset  ZeroCross=off
  " 1" : Gain  Gain=kneeFlexPosGain
  " 4" : Gain  Gain=kneeFlexSpeedGain
  Add : Sum  Inputs=+-
  Add1 : Sum  Inputs=-+
  Constant : Constant  Value=TargetLegAngleTripFlex
  Saturation : Saturate  UpperLimit=0  LowerLimit=-inf  ZeroCross=off
  tau : Outport  OutputWhenDisabled=reset  InitialOutput=0
  wires:
  Saturation/1 -> " 4"/1
  " 4"/1 -> Add1/1
  LegAngleSpeed/1 -> Saturation/1
  Leg Angle/1 -> Add/2
  Constant/1 -> Add/1
  Add1/1 -> tau/1
  Add/1 -> " 1"/1
  " 1"/1 -> Add1/2

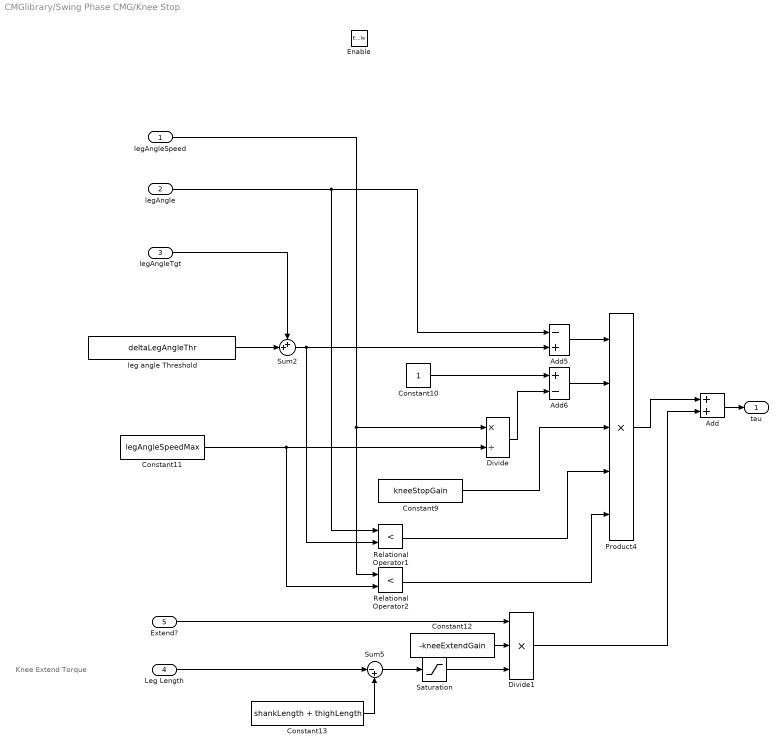
== system CMGlibrary/Swing Phase CMG/Knee Stop ==
  note: Knee Extend Torque
  legAngleSpeed : Inport
  legAngle : Inport  Port=2
  legAngleTgt : Inport  Port=3
  Leg Length : Inport  Port=4
  Extend? : Inport  Port=5
  Enable : EnablePort  StatesWhenEnabling=reset  ZeroCross=off
  Add : Sum
  Add5 : Sum  Inputs=-+
  Add6 : Sum  Inputs=+-
  Constant10 : Constant
  Constant11 : Constant  Value=legAngleSpeedMax
  Constant12 : Constant  Value=-kneeExtendGain
  Constant13 : Constant  Value=shankLength + thighLength
  Constant9 : Constant  Value=kneeStopGain
  Divide : Product  Inputs=*/
  Divide1 : Product  Inputs=***
  Product4 : Product  Inputs=5
  Relational Operator1 : RelationalOperator  Operator=<  OutDataTypeStr=boolean  ZeroCross=off  RndMeth=Nearest
  Relational Operator2 : RelationalOperator  Operator=<  OutDataTypeStr=boolean  ZeroCross=off  RndMeth=Nearest
  Saturation : Saturate  UpperLimit=inf  LowerLimit=0  ZeroCross=off
  Sum2 : Sum  Inputs=++|
  Sum5 : Sum  Inputs=|-+
  leg angle Threshold : Constant  Value=deltaLegAngleThr
  tau : Outport  OutputWhenDisabled=reset  InitialOutput=0
  wires:
  leg angle Threshold/1 -> Sum2/2
  Sum2/1 -> Add5/2, Relational Operator1/2
  Add5/1 -> Product4/1
  Constant9/1 -> Product4/3
  Constant11/1 -> Relational Operator2/2, Divide/2
  Add6/1 -> Product4/2
  Constant10/1 -> Add6/1
  Divide/1 -> Add6/2
  Relational Operator1/1 -> Product4/4
  Relational Operator2/1 -> Product4/5
  Product4/1 -> Add/1
  Constant12/1 -> Divide1/2
  Constant13/1 -> Sum5/2
  Sum5/1 -> Saturation/1
  Divide1/1 -> Add/2
  legAngleTgt/1 -> Sum2/1
  legAngle/1 -> Relational Operator1/1, Add5/1
  legAngleSpeed/1 -> Relational Operator2/1, Divide/1
  Leg Length/1 -> Sum5/1
  Extend?/1 -> Divide1/1
  Add/1 -> tau/1
  Saturation/1 -> Divide1/3

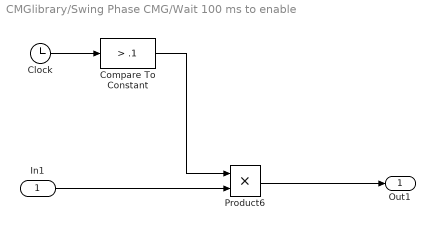
== system CMGlibrary/Swing Phase CMG/Wait 100 ms to enable ==
  In1 : Inport
  Clock : Clock
  Compare To Constant : simulink/Logic and Bit Operations/Compare To Constant  relop=>  const=.1  OutDataTypeStr=boolean  ZeroCross=off
  Product6 : Product
  Out1 : Outport
  wires:
  In1/1 -> Product6/2
  Compare To Constant/1 -> Product6/1
  Clock/1 -> Compare To Constant/1
  Product6/1 -> Out1/1

== stateflow chart CMGlibrary/Trip Detector/Chart ==
  settings: updateMethod=CONTINUOUS
  state Tripped_no_stance
    Active = 1;
    entry: start_time = time;
    exit: start_time = 0;
  state Tripped_but_stance
  state Stance
    Active = 0;
  Tripped_but_stance -> Tripped_no_stance : [~Stance]
  Tripped_no_stance -> Stance : [Stance && (time-start_time)>0.3]
  Stance -> Tripped_but_stance : [Tripped && time > 3 && ~trippedOnce]
  (default) -> Stance
  data: Active output double; Stance input; Tripped input; time input double; start_time local double; trippedOnce input double

== stateflow chart CMGlibrary/Swing Phase CMG/Chart ==
  settings: updateMethod=CONTINUOUS
  state KneeFlexion
    entry: flex = 1;
    exit: flex = 0;
  state KneeStopAndExtend
    entry: stop = 1;
    exit: stop = 0;
    state Extend
      entry: extend = 1;
      exit: extend = 0;
    state KneeStopOnly
    KneeStopOnly -> Extend : [true || legAngleSpeed >= 0]
    (default) -> KneeStopOnly
  KneeStopAndExtend -> KneeFlexion : [Stance]
  KneeFlexion -> KneeStopAndExtend : [(legLength < legLengthClr) && contraStance && ~Stance]
  (default) -> KneeStopAndExtend
  data: Stance input; contraStance input; legAngleSpeed input; legLength input; legLengthClr parameter; flex output double; stop output double; extend output double

== stateflow chart CMGlibrary/Swing Phase CMG/Chart1 ==
  settings: updateMethod=CONTINUOUS
  state KneeFlexion
    entry: flex = 1;
    exit: flex = 0;
  state KneeHoldStopAndExtend
    entry: hold = 1;
    exit: hold = 0;
    state KneeStopAndExtend
      entry: stop = 1;
      exit: stop = 0;
      state Extend
        entry: extend = 1;
        exit: extend = 0;
      state KneeStopOnly
      KneeStopOnly -> Extend : [legAngleSpeed >= 0]
      (default) -> KneeStopOnly
    state KneeHoldOnly
    KneeHoldOnly -> KneeStopAndExtend : [(legAngle < (legAngleTgt + ...
        | deltaLegAngleThr)) || Stance]
    (default) -> KneeHoldOnly
  KneeHoldStopAndExtend -> KneeFlexion : [Stance]
  KneeFlexion -> KneeHoldStopAndExtend : [(legLength < legLengthClr) && contraStance && ~Stance]
  (default) -> KneeHoldStopAndExtend
  data: Stance input; contraStance input; deltaLegAngleThr parameter; legAngle input; legAngleSpeed input; legAngleTgt input; legLength input; legLengthClr parameter; flex output double; hold output double; stop output double; extend output double
